simulink model "mfac"  (Simulink 7.4)
settings: Solver=ode45  StartTime=0.0  StopTime=100.0  RelTol=1e-3
settings Model: Creator=Administrator  LastModifiedBy=Administrator
settings DebuggingCC: SaveWithParameterizedLinksMsg=none

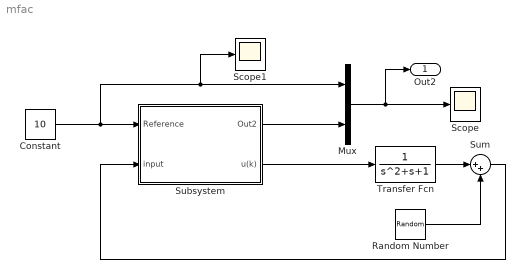
== system mfac ==
  Constant : Constant  Value=10  OutDataType=sfix(16)  OutScaling=2^0
  Mux : Mux  Inputs=2
  Random Number : RandomNumber  Variance=0.01  SampleTime=0.1
  Scope : Scope
      settings: TimeRange=20  YMin=-1  YMax=12  SampleInput=on  SampleTime=0.1
  Scope1 : Scope
  Subsystem : Subsystem  mask{c=0.1, d=0.016, t=0.01}
      mask prompts: c "Learning Rate"; d "Penality Factor"; t "Sampled Time"
      mask init:
      | c=0.07;
      | d=0.1;
      | t=1;
  Sum : Sum  Inputs=|++  OutDataType=fixdt(1, 16)  OutScaling=2^0
  Transfer Fcn : TransferFcn  Denominator=[1 1 1]
  Out2 : Outport  OutDataType=fixdt(1, 16)  OutScaling=2^0
  wires:
  Subsystem/1(Out2) -> Mux/2
  Transfer Fcn/1 -> Sum/1
  Sum/1 -> Subsystem/2(input)
  Mux/1 -> Out2/1, Scope/1
  Constant/1 -> Subsystem/1(Reference), Mux/1, Scope1/1
  Subsystem/2(u(k)) -> Transfer Fcn/1
  Random Number/1 -> Sum/2

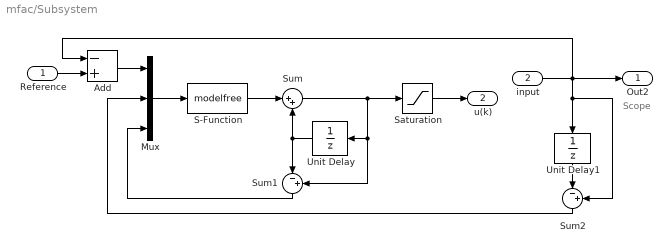
== system mfac/Subsystem ==
  note: Scope
  Reference : Inport  OutDataType=fixdt(1, 16)  OutScaling=2^0
  input : Inport  Port=2  OutDataType=fixdt(1, 16)  OutScaling=2^0
  Add : Sum  Inputs=-+  OutDataType=fixdt(1, 16)  OutScaling=2^-10
  Mux : Mux  Inputs=3
  S-Function : S-Function  FunctionName=modelfree  Parameters=c,d  EnableBusSupport=off
  Saturation : Saturate  UpperLimit=12  LowerLimit=0
  Sum : Sum  Inputs=|++  OutDataType=fixdt(1, 16)  OutScaling=2^0
  Sum1 : Sum  Inputs=|-+  OutDataType=fixdt(1, 16)  OutScaling=2^0
  Sum2 : Sum  Inputs=|-+  OutDataType=fixdt(1, 16)  OutScaling=2^0
  Unit Delay : UnitDelay  SampleTime=-1
  Unit Delay1 : UnitDelay  SampleTime=-1
  Out2 : Outport  OutDataType=fixdt(1, 16)  OutScaling=2^0
  u(k) : Outport  Port=2  OutDataType=fixdt(1, 16)  OutScaling=2^0
  wires:
  input/1 -> Out2/1, Add/1, Sum2/2, Unit Delay1/1
  Sum2/1 -> Mux/2
  Unit Delay1/1 -> Sum2/1
  Sum1/1 -> Mux/3
  Sum/1 -> Saturation/1, Sum1/2, Unit Delay/1
  S-Function/1 -> Sum/1
  Mux/1 -> S-Function/1
  Add/1 -> Mux/1
  Reference/1 -> Add/2
  Saturation/1 -> u(k)/1
  Unit Delay/1 -> Sum/2, Sum1/1
